simulink model "Allegato2"  (R2022b)
settings: Solver=VariableStepAuto  StartTime=0.0  StopTime=40  RelTol=1e-3
model workspace (MAT data in the model file):
  accthreshold = 0
libraries: SignalEditorBlockLib x1
settings Model: Creator=andre  LastModifiedBy=andre
settings SolverCC: ZeroCrossAlgorithm=Adaptive
settings DebuggingCC: IgnoredZcDiagnostic=none

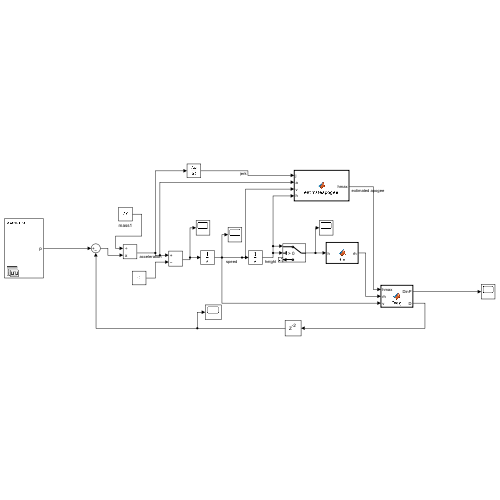
[thumbnail: Simulink's stored preview of the top-level diagram]
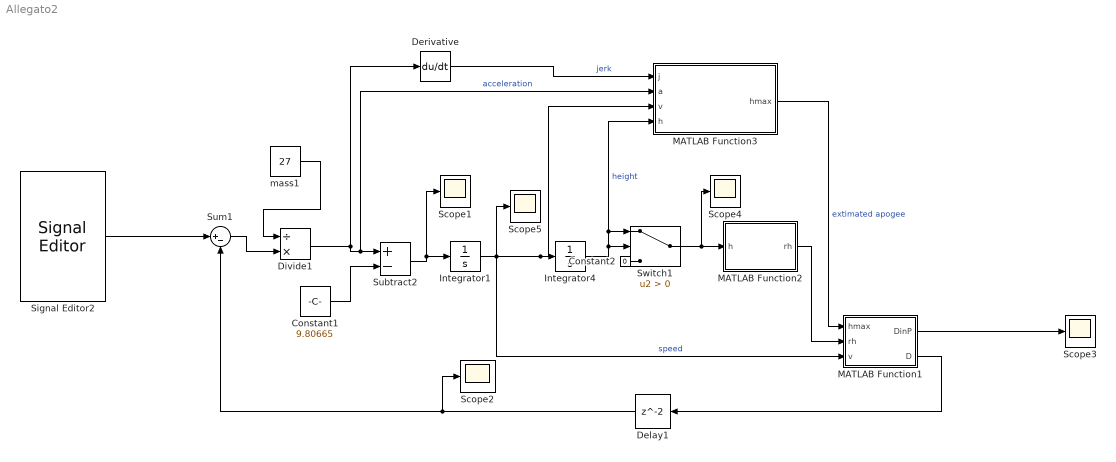
== system Allegato2 ==
  Constant1 : Constant  Value=9.80665
  Constant2 : Constant  Value=0
  Delay1 : Delay
  Derivative : Derivative
  Divide1 : Product  Inputs=/*
  Integrator1 : Integrator
  Integrator4 : Integrator
  MATLAB Function1 : MATLAB Function  TreatAsAtomicUnit=on
  MATLAB Function2 : MATLAB Function  TreatAsAtomicUnit=on
  MATLAB Function3 : MATLAB Function  TreatAsAtomicUnit=on
  Scope{1..5} (5 alike) : Scope
  Signal Editor2 : SignalEditorBlockLib/Signal Editor  FileName=C:\Users\andre\Desktop\ANDREA_STEFANI\Allegati\AeroTech_M2000R.mat  ActiveScenario=Scenario  ActiveSignal=p  IsBus=off  OutputBusObjectStr=Bus: BusObject  SampleTime=0  Interpolate=off  ZeroCross=off  OutputAfterFinalValue=Setting to zero  Unit=inherit  PreserveSignalName=on
  Subtract2 : Sum  Inputs=+-
  Sum1 : Sum  Inputs=|+-
  Switch1 : Switch  Criteria=u2 > Threshold  SaturateOnIntegerOverflow=off  InputSameDT=off
  mass1 : Constant  Value=27
  wires:
  MATLAB Function3/1(hmax) -> MATLAB Function1/1(hmax)  "extimated apogee"
  Subtract2/1 -> Scope1/1, Integrator1/1
  Integrator1/1 -> Scope5/1, MATLAB Function3/3(v), Integrator4/1, MATLAB Function1/3(v)  "speed"
  MATLAB Function2/1(rh) -> MATLAB Function1/2(rh)
  Switch1/1 -> Scope4/1, MATLAB Function2/1(h)
  Signal Editor2/1 -> Sum1/1
  mass1/1 -> Divide1/1
  Constant1/1 -> Subtract2/2
  MATLAB Function1/1(DinP) -> Scope3/1
  Sum1/1 -> Divide1/2
  MATLAB Function1/2(D) -> Delay1/1
  Integrator4/1 -> MATLAB Function3/4(h), Switch1/1, Switch1/2  "height"
  Delay1/1 -> Sum1/2, Scope2/1
  Divide1/1 -> Derivative/1, Subtract2/1, MATLAB Function3/2(a)  "acceleration"
  Constant2/1 -> Switch1/3
  Derivative/1 -> MATLAB Function3/1(j)  "jerk"

== matlab function Allegato2/MATLAB Function1 ==
  data: hmax input; rh input; v input; DinP output; D output
function [DinP, D]= Drag(hmax, rh, v)
S=pi*0.075^2;
DinP=0.5*rh*v^2;
if hmax>3000 && DinP<4*10^4 
    cd=0.85;
else
    cd=0.36;
end
D = DinP*S*cd;

== matlab function Allegato2/MATLAB Function2 ==
  data: h input; rh output
function rh = rho(h)
rh0=1.2250
g0=9.80665
M=0.0289644 %molar mass of air
R=8.3144598
T=288.15
rh = rh0*exp(-g0*M*h/(R*T));

== matlab function Allegato2/MATLAB Function3 ==
  data: j input; a input; v input; h input; hmax output
function hmax = estimateapogee(j, a, v, h)
H= zeros(10, 1);
for i = 1:10
    H(i) = h+v*i+1/2*a*i^2+1/6*j*i^3;
end
hmax1= max(H);
hmax=hmax1(1);
